simulink model "SPGF_FSK_0000_R2022b"  (R2022b)
settings: Solver=ode4  StartTime=0.0  StopTime=1.4  FixedStep=50e-6/50  RelTol=1e-3  EnableMultiTasking=on
undefined symbols (not defined in the file): D11, Delta
libraries: spsSeriesRLCBranchLib x1646, spsGroundLib x360, spsStairGeneratorLib x147, spsIdealSwitchLib x145, spsCurrentMeasurementLib x145, spsUniversalBridgeLib x76, spsThreePhaseSeriesRLCLoadLib x57, simulink x45, spsBistableLib x36, spsSequenceAnalyzerLib x31, spsThreePhaseParallelRLCLoadLib x20, spsThreePhaseTransformerTwoWindingsLib x20
(part 35 of 40)

== system SPGF_FSK_0000_R2022b/K2/fault/Arcing ==
  m : Inport
  Inter : Inport  Port=2
  Enable : EnablePort  StatesWhenEnabling=reset
  Abs3 : Abs  SaturateOnIntegerOverflow=off
  ArcStrV : Subsystem
  Bistable : spsBistableLib/Bistable  Qpriority=Set  ic=0  Ts=0
      settings: LibrarySourceBlock=sps_lib/Control/Bistable
  Constant1 : Constant  Value=TheoryOfArc
  Constant4 : Constant  Value=TheoryOfArc
  DTC_B : DataTypeConversion  OutDataTypeStr=boolean  SaturateOnIntegerOverflow=off  RndMeth=Floor
  DTC_D : DataTypeConversion  OutDataTypeStr=double  SaturateOnIntegerOverflow=off  RndMeth=Floor
  Demux : Demux  Outputs=2
  Fault A10 : Constant
  Fault A11 : Constant  Value=0
  Peters & Slepian : Subsystem
  Product : Product
  Relational Operator4 : RelationalOperator  OutDataTypeStr=boolean  InputSameDT=off
  SW_1 : MultiPortSwitch  DataPortForDefault=Additional data port  SaturateOnIntegerOverflow=off  InputSameDT=off
  SW_2 : Switch  Criteria=u2 > Threshold  Threshold=2  SaturateOnIntegerOverflow=off  InputSameDT=off
  Subsystem : Subsystem
  Terminator3 : Terminator
  Zero Crossing : Subsystem
  O : Outport  InitialOutput=[0]
  wires:
  Subsystem/1(O) -> Product/2
  Inter/1 -> [Inter]
  Relational Operator4/1 -> Product/1
  [Inter] -> Subsystem/1(I)
  Peters & Slepian/1(O) -> SW_2/1
  [I] -> Peters & Slepian/3(I)
  [Arc] -> Peters & Slepian/2(Arc)
  [I] -> Zero Crossing/1(I)
  Zero Crossing/1(O) -> SW_2/3, Peters & Slepian/1(ZC)  "Petersen"
  ArcStrV/1(Vset) -> Relational Operator4/2
  m/1 -> Demux/1
  Demux/2 -> [V]
  Demux/1 -> [I]
  Constant4/1 -> SW_2/2
  SW_2/1 -> DTC_B/1
  Abs3/1 -> Relational Operator4/1
  [V] -> Abs3/1
  DTC_D/1 -> SW_1/4, SW_1/3
  DTC_B/1 -> Bistable/2
  Bistable/2 -> Terminator3/1
  Product/1 -> [Arc], Bistable/1
  Bistable/1 -> DTC_D/1
  Fault A11/1 -> SW_1/5
  Fault A10/1 -> SW_1/2
  SW_1/1 -> O/1
  Constant1/1 -> SW_1/1

== system SPGF_FSK_0000_R2022b/K2/fault/Count Limiter ==
  I : Inport
  Counter : Subsystem  TreatAsAtomicUnit=on
  Fault A13 : Constant  Value=0
  Fault A3 : Constant
  Switch4 : Switch  Threshold=ArcingNumber  SaturateOnIntegerOverflow=off  InputSameDT=off
  Count : Outport
  O : Outport  Port=2
  wires:
  Counter/1(O) -> Count/1, Switch4/2
  Fault A13/1 -> Switch4/1
  Fault A3/1 -> Counter/1(I)
  I/1 -> Counter/Trigger, Switch4/3
  Switch4/1 -> O/1

== system SPGF_FSK_0000_R2022b/K2/fault/InitialPhaseCtrl ==
  m : Inport
  Enable : EnablePort  StatesWhenEnabling=reset
  Bistable : spsBistableLib/Bistable  Qpriority=Set  ic=0  Ts=0
      settings: LibrarySourceBlock=sps_lib/Control/Bistable
  Bistable1 : spsBistableLib/Bistable  Qpriority=Set  ic=0  Ts=0
      settings: LibrarySourceBlock=sps_lib/Control/Bistable
  Compare To Zero : simulink/Logic and Bit Operations/Compare To Zero  relop=~=  OutDataTypeStr=boolean
  Constant1 : Constant  Value=InitialPhaseCtrl
  DTC_D : DataTypeConversion  OutDataTypeStr=double  SaturateOnIntegerOverflow=off  RndMeth=Floor
  DTC_D1 : DataTypeConversion  OutDataTypeStr=double  SaturateOnIntegerOverflow=off  RndMeth=Floor
  DTC_D2 : DataTypeConversion  OutDataTypeStr=double  SaturateOnIntegerOverflow=off  RndMeth=Floor
  Demux : Demux  Outputs=2
  Fault A11 : Constant
  Hit Crossing : HitCross
  Off Delay : spsOffDelayLib/Off Delay  DelayType=On delay  delay=FaultDelay  ic=0  Ts=0
      settings: LibrarySourceBlock=sps_lib/Control/Off Delay
  Product1 : Product
  SW_1 : MultiPortSwitch  Inputs=2  SaturateOnIntegerOverflow=off  InputSameDT=off
  Terminator : Terminator
  Terminator1 : Terminator
  Terminator3 : Terminator
  O : Outport  InitialOutput=[0]
  wires:
  Bistable1/2 -> Terminator1/1
  DTC_D1/1 -> Product1/2
  Bistable1/1 -> DTC_D1/1
  DTC_D/1 -> SW_1/2
  Fault A11/1 -> SW_1/3
  Off Delay/1 -> Bistable/1
  Bistable/1 -> DTC_D/1
  Bistable/2 -> Terminator3/1
  Constant1/1 -> SW_1/1
  SW_1/1 -> O/1
  Demux/1 -> Terminator/1
  Demux/2 -> [V]
  m/1 -> Demux/1
  Product1/1 -> Off Delay/1
  [V] -> Hit Crossing/1, Compare To Zero/1
  Compare To Zero/1 -> DTC_D2/1
  Hit Crossing/1 -> Bistable1/1
  DTC_D2/1 -> Product1/1

== system SPGF_FSK_0000_R2022b/K2/fault/Interruption ==
  Band-Limited White Noise1 : simulink/Sources/Band-Limited White Noise  Cov=[.1]  Ts=NoiseSampleTime  seed=NoiseSeed
  Constant1 : Constant  Value=TypeOfPause
  Fault A10 : Constant
  Fault A11 : Constant  Value=0
  Multiport Switch : MultiPortSwitch  Inputs=4  DataPortForDefault=Additional data port  SaturateOnIntegerOverflow=off  InputSameDT=off
  Pulse Generator : DiscretePulseGenerator  PulseType=Time based  Period=PulsePeriod  PulseWidth=PulseWidth  PhaseDelay=PhaseDelay
  Rate Transition1 : RateTransition
  Saturation1 : Saturate  UpperLimit=1  LowerLimit=0
  Sign1 : Signum
  "Stair Generator " : spsStairGeneratorLib/Stair Generator  t=SwitchTimes  e=SwitchStatus  Ts=0
  O : Outport
  wires:
  Band-Limited White Noise1/1 -> Sign1/1
  "Stair Generator "/1 -> Multiport Switch/5
  Rate Transition1/1 -> Multiport Switch/3
  Saturation1/1 -> Rate Transition1/1
  Pulse Generator/1 -> Multiport Switch/4
  Constant1/1 -> Multiport Switch/1
  Sign1/1 -> Saturation1/1
  Fault A11/1 -> Multiport Switch/6
  Fault A10/1 -> Multiport Switch/2
  Multiport Switch/1 -> O/1

== system SPGF_FSK_0000_R2022b/K2/fault/Time Delay ==
  Count : Inport
  Control : Inport  Port=2
  Constant1 : Constant  Value=TimeDelay
  Constant3 : Constant  Value=0
  Memory : Memory
  SC_Time5 : Subsystem
      mask Display: disp('Delay');
  SW_Num : Switch  Threshold=ArcingNumber  SaturateOnIntegerOverflow=off  InputSameDT=off
  Selector : Selector  IndexMode=Zero-based  InputPortWidth=ArcingNumber  IndexOptions=Index vector (port)  Indices=[1 4]  OutputSizes=1
  O : Outport
  wires:
  Memory/1 -> SW_Num/3
  Control/1 -> SC_Time5/1(Control)
  SC_Time5/1(Out) -> O/1
  Count/1 -> SW_Num/2, Memory/1
  Constant1/1 -> Selector/1
  Selector/1 -> SC_Time5/2(TimeDelay)
  Constant3/1 -> SW_Num/1
  SW_Num/1 -> Selector/2

== system SPGF_FSK_0000_R2022b/K3/fault/Arcing ==
  m : Inport
  Inter : Inport  Port=2
  Enable : EnablePort  StatesWhenEnabling=reset
  Abs3 : Abs  SaturateOnIntegerOverflow=off
  ArcStrV : Subsystem
  Bistable : spsBistableLib/Bistable  Qpriority=Set  ic=0  Ts=0
      settings: LibrarySourceBlock=sps_lib/Control/Bistable
  Constant1 : Constant  Value=TheoryOfArc
  Constant4 : Constant  Value=TheoryOfArc
  DTC_B : DataTypeConversion  OutDataTypeStr=boolean  SaturateOnIntegerOverflow=off  RndMeth=Floor
  DTC_D : DataTypeConversion  OutDataTypeStr=double  SaturateOnIntegerOverflow=off  RndMeth=Floor
  Demux : Demux  Outputs=2
  Fault A10 : Constant
  Fault A11 : Constant  Value=0
  Peters & Slepian : Subsystem
  Product : Product
  Relational Operator4 : RelationalOperator  OutDataTypeStr=boolean  InputSameDT=off
  SW_1 : MultiPortSwitch  DataPortForDefault=Additional data port  SaturateOnIntegerOverflow=off  InputSameDT=off
  SW_2 : Switch  Criteria=u2 > Threshold  Threshold=2  SaturateOnIntegerOverflow=off  InputSameDT=off
  Subsystem : Subsystem
  Terminator3 : Terminator
  Zero Crossing : Subsystem
  O : Outport  InitialOutput=[0]
  wires:
  Subsystem/1(O) -> Product/2
  Inter/1 -> [Inter]
  Relational Operator4/1 -> Product/1
  [Inter] -> Subsystem/1(I)
  Peters & Slepian/1(O) -> SW_2/1
  [I] -> Peters & Slepian/3(I)
  [Arc] -> Peters & Slepian/2(Arc)
  [I] -> Zero Crossing/1(I)
  Zero Crossing/1(O) -> SW_2/3, Peters & Slepian/1(ZC)  "Petersen"
  ArcStrV/1(Vset) -> Relational Operator4/2
  m/1 -> Demux/1
  Demux/2 -> [V]
  Demux/1 -> [I]
  Constant4/1 -> SW_2/2
  SW_2/1 -> DTC_B/1
  Abs3/1 -> Relational Operator4/1
  [V] -> Abs3/1
  DTC_D/1 -> SW_1/4, SW_1/3
  DTC_B/1 -> Bistable/2
  Bistable/2 -> Terminator3/1
  Product/1 -> [Arc], Bistable/1
  Bistable/1 -> DTC_D/1
  Fault A11/1 -> SW_1/5
  Fault A10/1 -> SW_1/2
  SW_1/1 -> O/1
  Constant1/1 -> SW_1/1

== system SPGF_FSK_0000_R2022b/K3/fault/Count Limiter ==
  I : Inport
  Counter : Subsystem  TreatAsAtomicUnit=on
  Fault A13 : Constant  Value=0
  Fault A3 : Constant
  Switch4 : Switch  Threshold=ArcingNumber  SaturateOnIntegerOverflow=off  InputSameDT=off
  Count : Outport
  O : Outport  Port=2
  wires:
  Counter/1(O) -> Count/1, Switch4/2
  Fault A13/1 -> Switch4/1
  Fault A3/1 -> Counter/1(I)
  I/1 -> Counter/Trigger, Switch4/3
  Switch4/1 -> O/1

== system SPGF_FSK_0000_R2022b/K3/fault/InitialPhaseCtrl ==
  m : Inport
  Enable : EnablePort  StatesWhenEnabling=reset
  Bistable : spsBistableLib/Bistable  Qpriority=Set  ic=0  Ts=0
      settings: LibrarySourceBlock=sps_lib/Control/Bistable
  Bistable1 : spsBistableLib/Bistable  Qpriority=Set  ic=0  Ts=0
      settings: LibrarySourceBlock=sps_lib/Control/Bistable
  Compare To Zero : simulink/Logic and Bit Operations/Compare To Zero  relop=~=  OutDataTypeStr=boolean
  Constant1 : Constant  Value=InitialPhaseCtrl
  DTC_D : DataTypeConversion  OutDataTypeStr=double  SaturateOnIntegerOverflow=off  RndMeth=Floor
  DTC_D1 : DataTypeConversion  OutDataTypeStr=double  SaturateOnIntegerOverflow=off  RndMeth=Floor
  DTC_D2 : DataTypeConversion  OutDataTypeStr=double  SaturateOnIntegerOverflow=off  RndMeth=Floor
  Demux : Demux  Outputs=2
  Fault A11 : Constant
  Hit Crossing : HitCross
  Off Delay : spsOffDelayLib/Off Delay  DelayType=On delay  delay=FaultDelay  ic=0  Ts=0
      settings: LibrarySourceBlock=sps_lib/Control/Off Delay
  Product1 : Product
  SW_1 : MultiPortSwitch  Inputs=2  SaturateOnIntegerOverflow=off  InputSameDT=off
  Terminator : Terminator
  Terminator1 : Terminator
  Terminator3 : Terminator
  O : Outport  InitialOutput=[0]
  wires:
  Bistable1/2 -> Terminator1/1
  DTC_D1/1 -> Product1/2
  Bistable1/1 -> DTC_D1/1
  DTC_D/1 -> SW_1/2
  Fault A11/1 -> SW_1/3
  Off Delay/1 -> Bistable/1
  Bistable/1 -> DTC_D/1
  Bistable/2 -> Terminator3/1
  Constant1/1 -> SW_1/1
  SW_1/1 -> O/1
  Demux/1 -> Terminator/1
  Demux/2 -> [V]
  m/1 -> Demux/1
  Product1/1 -> Off Delay/1
  [V] -> Hit Crossing/1, Compare To Zero/1
  Compare To Zero/1 -> DTC_D2/1
  Hit Crossing/1 -> Bistable1/1
  DTC_D2/1 -> Product1/1

== system SPGF_FSK_0000_R2022b/K3/fault/Interruption ==
  Band-Limited White Noise1 : simulink/Sources/Band-Limited White Noise  Cov=[.1]  Ts=NoiseSampleTime  seed=NoiseSeed
  Constant1 : Constant  Value=TypeOfPause
  Fault A10 : Constant
  Fault A11 : Constant  Value=0
  Multiport Switch : MultiPortSwitch  Inputs=4  DataPortForDefault=Additional data port  SaturateOnIntegerOverflow=off  InputSameDT=off
  Pulse Generator : DiscretePulseGenerator  PulseType=Time based  Period=PulsePeriod  PulseWidth=PulseWidth  PhaseDelay=PhaseDelay
  Rate Transition1 : RateTransition
  Saturation1 : Saturate  UpperLimit=1  LowerLimit=0
  Sign1 : Signum
  "Stair Generator " : spsStairGeneratorLib/Stair Generator  t=SwitchTimes  e=SwitchStatus  Ts=0
  O : Outport
  wires:
  Band-Limited White Noise1/1 -> Sign1/1
  "Stair Generator "/1 -> Multiport Switch/5
  Rate Transition1/1 -> Multiport Switch/3
  Saturation1/1 -> Rate Transition1/1
  Pulse Generator/1 -> Multiport Switch/4
  Constant1/1 -> Multiport Switch/1
  Sign1/1 -> Saturation1/1
  Fault A11/1 -> Multiport Switch/6
  Fault A10/1 -> Multiport Switch/2
  Multiport Switch/1 -> O/1

== system SPGF_FSK_0000_R2022b/K3/fault/Time Delay ==
  Count : Inport
  Control : Inport  Port=2
  Constant1 : Constant  Value=TimeDelay
  Constant3 : Constant  Value=0
  Memory : Memory
  SC_Time5 : Subsystem
      mask Display: disp('Delay');
  SW_Num : Switch  Threshold=ArcingNumber  SaturateOnIntegerOverflow=off  InputSameDT=off
  Selector : Selector  IndexMode=Zero-based  InputPortWidth=ArcingNumber  IndexOptions=Index vector (port)  Indices=[1 4]  OutputSizes=1
  O : Outport
  wires:
  Memory/1 -> SW_Num/3
  Control/1 -> SC_Time5/1(Control)
  SC_Time5/1(Out) -> O/1
  Count/1 -> SW_Num/2, Memory/1
  Constant1/1 -> Selector/1
  Selector/1 -> SC_Time5/2(TimeDelay)
  Constant3/1 -> SW_Num/1
  SW_Num/1 -> Selector/2

== system SPGF_FSK_0000_R2022b/K4/fault/Arcing ==
  m : Inport
  Inter : Inport  Port=2
  Enable : EnablePort  StatesWhenEnabling=reset
  Abs3 : Abs  SaturateOnIntegerOverflow=off
  ArcStrV : Subsystem
  Bistable : spsBistableLib/Bistable  Qpriority=Set  ic=0  Ts=0
      settings: LibrarySourceBlock=sps_lib/Control/Bistable
  Constant1 : Constant  Value=TheoryOfArc
  Constant4 : Constant  Value=TheoryOfArc
  DTC_B : DataTypeConversion  OutDataTypeStr=boolean  SaturateOnIntegerOverflow=off  RndMeth=Floor
  DTC_D : DataTypeConversion  OutDataTypeStr=double  SaturateOnIntegerOverflow=off  RndMeth=Floor
  Demux : Demux  Outputs=2
  Fault A10 : Constant
  Fault A11 : Constant  Value=0
  Peters & Slepian : Subsystem
  Product : Product
  Relational Operator4 : RelationalOperator  OutDataTypeStr=boolean  InputSameDT=off
  SW_1 : MultiPortSwitch  DataPortForDefault=Additional data port  SaturateOnIntegerOverflow=off  InputSameDT=off
  SW_2 : Switch  Criteria=u2 > Threshold  Threshold=2  SaturateOnIntegerOverflow=off  InputSameDT=off
  Subsystem : Subsystem
  Terminator3 : Terminator
  Zero Crossing : Subsystem
  O : Outport  InitialOutput=[0]
  wires:
  Subsystem/1(O) -> Product/2
  Inter/1 -> [Inter]
  Relational Operator4/1 -> Product/1
  [Inter] -> Subsystem/1(I)
  Peters & Slepian/1(O) -> SW_2/1
  [I] -> Peters & Slepian/3(I)
  [Arc] -> Peters & Slepian/2(Arc)
  [I] -> Zero Crossing/1(I)
  Zero Crossing/1(O) -> SW_2/3, Peters & Slepian/1(ZC)  "Petersen"
  ArcStrV/1(Vset) -> Relational Operator4/2
  m/1 -> Demux/1
  Demux/2 -> [V]
  Demux/1 -> [I]
  Constant4/1 -> SW_2/2
  SW_2/1 -> DTC_B/1
  Abs3/1 -> Relational Operator4/1
  [V] -> Abs3/1
  DTC_D/1 -> SW_1/4, SW_1/3
  DTC_B/1 -> Bistable/2
  Bistable/2 -> Terminator3/1
  Product/1 -> [Arc], Bistable/1
  Bistable/1 -> DTC_D/1
  Fault A11/1 -> SW_1/5
  Fault A10/1 -> SW_1/2
  SW_1/1 -> O/1
  Constant1/1 -> SW_1/1

== system SPGF_FSK_0000_R2022b/K4/fault/Count Limiter ==
  I : Inport
  Counter : Subsystem  TreatAsAtomicUnit=on
  Fault A13 : Constant  Value=0
  Fault A3 : Constant
  Switch4 : Switch  Threshold=ArcingNumber  SaturateOnIntegerOverflow=off  InputSameDT=off
  Count : Outport
  O : Outport  Port=2
  wires:
  Counter/1(O) -> Count/1, Switch4/2
  Fault A13/1 -> Switch4/1
  Fault A3/1 -> Counter/1(I)
  I/1 -> Counter/Trigger, Switch4/3
  Switch4/1 -> O/1

== system SPGF_FSK_0000_R2022b/K4/fault/InitialPhaseCtrl ==
  m : Inport
  Enable : EnablePort  StatesWhenEnabling=reset
  Bistable : spsBistableLib/Bistable  Qpriority=Set  ic=0  Ts=0
      settings: LibrarySourceBlock=sps_lib/Control/Bistable
  Bistable1 : spsBistableLib/Bistable  Qpriority=Set  ic=0  Ts=0
      settings: LibrarySourceBlock=sps_lib/Control/Bistable
  Compare To Zero : simulink/Logic and Bit Operations/Compare To Zero  relop=~=  OutDataTypeStr=boolean
  Constant1 : Constant  Value=InitialPhaseCtrl
  DTC_D : DataTypeConversion  OutDataTypeStr=double  SaturateOnIntegerOverflow=off  RndMeth=Floor
  DTC_D1 : DataTypeConversion  OutDataTypeStr=double  SaturateOnIntegerOverflow=off  RndMeth=Floor
  DTC_D2 : DataTypeConversion  OutDataTypeStr=double  SaturateOnIntegerOverflow=off  RndMeth=Floor
  Demux : Demux  Outputs=2
  Fault A11 : Constant
  Hit Crossing : HitCross
  Off Delay : spsOffDelayLib/Off Delay  DelayType=On delay  delay=FaultDelay  ic=0  Ts=0
      settings: LibrarySourceBlock=sps_lib/Control/Off Delay
  Product1 : Product
  SW_1 : MultiPortSwitch  Inputs=2  SaturateOnIntegerOverflow=off  InputSameDT=off
  Terminator : Terminator
  Terminator1 : Terminator
  Terminator3 : Terminator
  O : Outport  InitialOutput=[0]
  wires:
  Bistable1/2 -> Terminator1/1
  DTC_D1/1 -> Product1/2
  Bistable1/1 -> DTC_D1/1
  DTC_D/1 -> SW_1/2
  Fault A11/1 -> SW_1/3
  Off Delay/1 -> Bistable/1
  Bistable/1 -> DTC_D/1
  Bistable/2 -> Terminator3/1
  Constant1/1 -> SW_1/1
  SW_1/1 -> O/1
  Demux/1 -> Terminator/1
  Demux/2 -> [V]
  m/1 -> Demux/1
  Product1/1 -> Off Delay/1
  [V] -> Hit Crossing/1, Compare To Zero/1
  Compare To Zero/1 -> DTC_D2/1
  Hit Crossing/1 -> Bistable1/1
  DTC_D2/1 -> Product1/1

== system SPGF_FSK_0000_R2022b/K4/fault/Interruption ==
  Band-Limited White Noise1 : simulink/Sources/Band-Limited White Noise  Cov=[.1]  Ts=NoiseSampleTime  seed=NoiseSeed
  Constant1 : Constant  Value=TypeOfPause
  Fault A10 : Constant
  Fault A11 : Constant  Value=0
  Multiport Switch : MultiPortSwitch  Inputs=4  DataPortForDefault=Additional data port  SaturateOnIntegerOverflow=off  InputSameDT=off
  Pulse Generator : DiscretePulseGenerator  PulseType=Time based  Period=PulsePeriod  PulseWidth=PulseWidth  PhaseDelay=PhaseDelay
  Rate Transition1 : RateTransition
  Saturation1 : Saturate  UpperLimit=1  LowerLimit=0
  Sign1 : Signum
  "Stair Generator " : spsStairGeneratorLib/Stair Generator  t=SwitchTimes  e=SwitchStatus  Ts=0
  O : Outport
  wires:
  Band-Limited White Noise1/1 -> Sign1/1
  "Stair Generator "/1 -> Multiport Switch/5
  Rate Transition1/1 -> Multiport Switch/3
  Saturation1/1 -> Rate Transition1/1
  Pulse Generator/1 -> Multiport Switch/4
  Constant1/1 -> Multiport Switch/1
  Sign1/1 -> Saturation1/1
  Fault A11/1 -> Multiport Switch/6
  Fault A10/1 -> Multiport Switch/2
  Multiport Switch/1 -> O/1

== system SPGF_FSK_0000_R2022b/K4/fault/Time Delay ==
  Count : Inport
  Control : Inport  Port=2
  Constant1 : Constant  Value=TimeDelay
  Constant3 : Constant  Value=0
  Memory : Memory
  SC_Time5 : Subsystem
      mask Display: disp('Delay');
  SW_Num : Switch  Threshold=ArcingNumber  SaturateOnIntegerOverflow=off  InputSameDT=off
  Selector : Selector  IndexMode=Zero-based  InputPortWidth=ArcingNumber  IndexOptions=Index vector (port)  Indices=[1 4]  OutputSizes=1
  O : Outport
  wires:
  Memory/1 -> SW_Num/3
  Control/1 -> SC_Time5/1(Control)
  SC_Time5/1(Out) -> O/1
  Count/1 -> SW_Num/2, Memory/1
  Constant1/1 -> Selector/1
  Selector/1 -> SC_Time5/2(TimeDelay)
  Constant3/1 -> SW_Num/1
  SW_Num/1 -> Selector/2

== system SPGF_FSK_0000_R2022b/K5/fault/Arcing ==
  m : Inport
  Inter : Inport  Port=2
  Enable : EnablePort  StatesWhenEnabling=reset
  Abs3 : Abs  SaturateOnIntegerOverflow=off
  ArcStrV : Subsystem
  Bistable : spsBistableLib/Bistable  Qpriority=Set  ic=0  Ts=0
      settings: LibrarySourceBlock=sps_lib/Control/Bistable
  Constant1 : Constant  Value=TheoryOfArc
  Constant4 : Constant  Value=TheoryOfArc
  DTC_B : DataTypeConversion  OutDataTypeStr=boolean  SaturateOnIntegerOverflow=off  RndMeth=Floor
  DTC_D : DataTypeConversion  OutDataTypeStr=double  SaturateOnIntegerOverflow=off  RndMeth=Floor
  Demux : Demux  Outputs=2
  Fault A10 : Constant
  Fault A11 : Constant  Value=0
  Peters & Slepian : Subsystem
  Product : Product
  Relational Operator4 : RelationalOperator  OutDataTypeStr=boolean  InputSameDT=off
  SW_1 : MultiPortSwitch  DataPortForDefault=Additional data port  SaturateOnIntegerOverflow=off  InputSameDT=off
  SW_2 : Switch  Criteria=u2 > Threshold  Threshold=2  SaturateOnIntegerOverflow=off  InputSameDT=off
  Subsystem : Subsystem
  Terminator3 : Terminator
  Zero Crossing : Subsystem
  O : Outport  InitialOutput=[0]
  wires:
  Subsystem/1(O) -> Product/2
  Inter/1 -> [Inter]
  Relational Operator4/1 -> Product/1
  [Inter] -> Subsystem/1(I)
  Peters & Slepian/1(O) -> SW_2/1
  [I] -> Peters & Slepian/3(I)
  [Arc] -> Peters & Slepian/2(Arc)
  [I] -> Zero Crossing/1(I)
  Zero Crossing/1(O) -> SW_2/3, Peters & Slepian/1(ZC)  "Petersen"
  ArcStrV/1(Vset) -> Relational Operator4/2
  m/1 -> Demux/1
  Demux/2 -> [V]
  Demux/1 -> [I]
  Constant4/1 -> SW_2/2
  SW_2/1 -> DTC_B/1
  Abs3/1 -> Relational Operator4/1
  [V] -> Abs3/1
  DTC_D/1 -> SW_1/4, SW_1/3
  DTC_B/1 -> Bistable/2
  Bistable/2 -> Terminator3/1
  Product/1 -> [Arc], Bistable/1
  Bistable/1 -> DTC_D/1
  Fault A11/1 -> SW_1/5
  Fault A10/1 -> SW_1/2
  SW_1/1 -> O/1
  Constant1/1 -> SW_1/1

== system SPGF_FSK_0000_R2022b/K5/fault/Count Limiter ==
  I : Inport
  Counter : Subsystem  TreatAsAtomicUnit=on
  Fault A13 : Constant  Value=0
  Fault A3 : Constant
  Switch4 : Switch  Threshold=ArcingNumber  SaturateOnIntegerOverflow=off  InputSameDT=off
  Count : Outport
  O : Outport  Port=2
  wires:
  Counter/1(O) -> Count/1, Switch4/2
  Fault A13/1 -> Switch4/1
  Fault A3/1 -> Counter/1(I)
  I/1 -> Counter/Trigger, Switch4/3
  Switch4/1 -> O/1

== system SPGF_FSK_0000_R2022b/K5/fault/InitialPhaseCtrl ==
  m : Inport
  Enable : EnablePort  StatesWhenEnabling=reset
  Bistable : spsBistableLib/Bistable  Qpriority=Set  ic=0  Ts=0
      settings: LibrarySourceBlock=sps_lib/Control/Bistable
  Bistable1 : spsBistableLib/Bistable  Qpriority=Set  ic=0  Ts=0
      settings: LibrarySourceBlock=sps_lib/Control/Bistable
  Compare To Zero : simulink/Logic and Bit Operations/Compare To Zero  relop=~=  OutDataTypeStr=boolean
  Constant1 : Constant  Value=InitialPhaseCtrl
  DTC_D : DataTypeConversion  OutDataTypeStr=double  SaturateOnIntegerOverflow=off  RndMeth=Floor
  DTC_D1 : DataTypeConversion  OutDataTypeStr=double  SaturateOnIntegerOverflow=off  RndMeth=Floor
  DTC_D2 : DataTypeConversion  OutDataTypeStr=double  SaturateOnIntegerOverflow=off  RndMeth=Floor
  Demux : Demux  Outputs=2
  Fault A11 : Constant
  Hit Crossing : HitCross
  Off Delay : spsOffDelayLib/Off Delay  DelayType=On delay  delay=FaultDelay  ic=0  Ts=0
      settings: LibrarySourceBlock=sps_lib/Control/Off Delay
  Product1 : Product
  SW_1 : MultiPortSwitch  Inputs=2  SaturateOnIntegerOverflow=off  InputSameDT=off
  Terminator : Terminator
  Terminator1 : Terminator
  Terminator3 : Terminator
  O : Outport  InitialOutput=[0]
  wires:
  Bistable1/2 -> Terminator1/1
  DTC_D1/1 -> Product1/2
  Bistable1/1 -> DTC_D1/1
  DTC_D/1 -> SW_1/2
  Fault A11/1 -> SW_1/3
  Off Delay/1 -> Bistable/1
  Bistable/1 -> DTC_D/1
  Bistable/2 -> Terminator3/1
  Constant1/1 -> SW_1/1
  SW_1/1 -> O/1
  Demux/1 -> Terminator/1
  Demux/2 -> [V]
  m/1 -> Demux/1
  Product1/1 -> Off Delay/1
  [V] -> Hit Crossing/1, Compare To Zero/1
  Compare To Zero/1 -> DTC_D2/1
  Hit Crossing/1 -> Bistable1/1
  DTC_D2/1 -> Product1/1

== system SPGF_FSK_0000_R2022b/K5/fault/Interruption ==
  Band-Limited White Noise1 : simulink/Sources/Band-Limited White Noise  Cov=[.1]  Ts=NoiseSampleTime  seed=NoiseSeed
  Constant1 : Constant  Value=TypeOfPause
  Fault A10 : Constant
  Fault A11 : Constant  Value=0
  Multiport Switch : MultiPortSwitch  Inputs=4  DataPortForDefault=Additional data port  SaturateOnIntegerOverflow=off  InputSameDT=off
  Pulse Generator : DiscretePulseGenerator  PulseType=Time based  Period=PulsePeriod  PulseWidth=PulseWidth  PhaseDelay=PhaseDelay
  Rate Transition1 : RateTransition
  Saturation1 : Saturate  UpperLimit=1  LowerLimit=0
  Sign1 : Signum
  "Stair Generator " : spsStairGeneratorLib/Stair Generator  t=SwitchTimes  e=SwitchStatus  Ts=0
  O : Outport
  wires:
  Band-Limited White Noise1/1 -> Sign1/1
  "Stair Generator "/1 -> Multiport Switch/5
  Rate Transition1/1 -> Multiport Switch/3
  Saturation1/1 -> Rate Transition1/1
  Pulse Generator/1 -> Multiport Switch/4
  Constant1/1 -> Multiport Switch/1
  Sign1/1 -> Saturation1/1
  Fault A11/1 -> Multiport Switch/6
  Fault A10/1 -> Multiport Switch/2
  Multiport Switch/1 -> O/1

== system SPGF_FSK_0000_R2022b/K5/fault/Time Delay ==
  Count : Inport
  Control : Inport  Port=2
  Constant1 : Constant  Value=TimeDelay
  Constant3 : Constant  Value=0
  Memory : Memory
  SC_Time5 : Subsystem
      mask Display: disp('Delay');
  SW_Num : Switch  Threshold=ArcingNumber  SaturateOnIntegerOverflow=off  InputSameDT=off
  Selector : Selector  IndexMode=Zero-based  InputPortWidth=ArcingNumber  IndexOptions=Index vector (port)  Indices=[1 4]  OutputSizes=1
  O : Outport
  wires:
  Memory/1 -> SW_Num/3
  Control/1 -> SC_Time5/1(Control)
  SC_Time5/1(Out) -> O/1
  Count/1 -> SW_Num/2, Memory/1
  Constant1/1 -> Selector/1
  Selector/1 -> SC_Time5/2(TimeDelay)
  Constant3/1 -> SW_Num/1
  SW_Num/1 -> Selector/2

== system SPGF_FSK_0000_R2022b/K6/fault/Arcing ==
  m : Inport
  Inter : Inport  Port=2
  Enable : EnablePort  StatesWhenEnabling=reset
  Abs3 : Abs  SaturateOnIntegerOverflow=off
  ArcStrV : Subsystem
  Bistable : spsBistableLib/Bistable  Qpriority=Set  ic=0  Ts=0
      settings: LibrarySourceBlock=sps_lib/Control/Bistable
  Constant1 : Constant  Value=TheoryOfArc
  Constant4 : Constant  Value=TheoryOfArc
  DTC_B : DataTypeConversion  OutDataTypeStr=boolean  SaturateOnIntegerOverflow=off  RndMeth=Floor
  DTC_D : DataTypeConversion  OutDataTypeStr=double  SaturateOnIntegerOverflow=off  RndMeth=Floor
  Demux : Demux  Outputs=2
  Fault A10 : Constant
  Fault A11 : Constant  Value=0
  Peters & Slepian : Subsystem
  Product : Product
  Relational Operator4 : RelationalOperator  OutDataTypeStr=boolean  InputSameDT=off
  SW_1 : MultiPortSwitch  DataPortForDefault=Additional data port  SaturateOnIntegerOverflow=off  InputSameDT=off
  SW_2 : Switch  Criteria=u2 > Threshold  Threshold=2  SaturateOnIntegerOverflow=off  InputSameDT=off
  Subsystem : Subsystem
  Terminator3 : Terminator
  Zero Crossing : Subsystem
  O : Outport  InitialOutput=[0]
  wires:
  Subsystem/1(O) -> Product/2
  Inter/1 -> [Inter]
  Relational Operator4/1 -> Product/1
  [Inter] -> Subsystem/1(I)
  Peters & Slepian/1(O) -> SW_2/1
  [I] -> Peters & Slepian/3(I)
  [Arc] -> Peters & Slepian/2(Arc)
  [I] -> Zero Crossing/1(I)
  Zero Crossing/1(O) -> SW_2/3, Peters & Slepian/1(ZC)  "Petersen"
  ArcStrV/1(Vset) -> Relational Operator4/2
  m/1 -> Demux/1
  Demux/2 -> [V]
  Demux/1 -> [I]
  Constant4/1 -> SW_2/2
  SW_2/1 -> DTC_B/1
  Abs3/1 -> Relational Operator4/1
  [V] -> Abs3/1
  DTC_D/1 -> SW_1/4, SW_1/3
  DTC_B/1 -> Bistable/2
  Bistable/2 -> Terminator3/1
  Product/1 -> [Arc], Bistable/1
  Bistable/1 -> DTC_D/1
  Fault A11/1 -> SW_1/5
  Fault A10/1 -> SW_1/2
  SW_1/1 -> O/1
  Constant1/1 -> SW_1/1

== system SPGF_FSK_0000_R2022b/K6/fault/Count Limiter ==
  I : Inport
  Counter : Subsystem  TreatAsAtomicUnit=on
  Fault A13 : Constant  Value=0
  Fault A3 : Constant
  Switch4 : Switch  Threshold=ArcingNumber  SaturateOnIntegerOverflow=off  InputSameDT=off
  Count : Outport
  O : Outport  Port=2
  wires:
  Counter/1(O) -> Count/1, Switch4/2
  Fault A13/1 -> Switch4/1
  Fault A3/1 -> Counter/1(I)
  I/1 -> Counter/Trigger, Switch4/3
  Switch4/1 -> O/1

== system SPGF_FSK_0000_R2022b/K6/fault/InitialPhaseCtrl ==
  m : Inport
  Enable : EnablePort  StatesWhenEnabling=reset
  Bistable : spsBistableLib/Bistable  Qpriority=Set  ic=0  Ts=0
      settings: LibrarySourceBlock=sps_lib/Control/Bistable
  Bistable1 : spsBistableLib/Bistable  Qpriority=Set  ic=0  Ts=0
      settings: LibrarySourceBlock=sps_lib/Control/Bistable
  Compare To Zero : simulink/Logic and Bit Operations/Compare To Zero  relop=~=  OutDataTypeStr=boolean
  Constant1 : Constant  Value=InitialPhaseCtrl
  DTC_D : DataTypeConversion  OutDataTypeStr=double  SaturateOnIntegerOverflow=off  RndMeth=Floor
  DTC_D1 : DataTypeConversion  OutDataTypeStr=double  SaturateOnIntegerOverflow=off  RndMeth=Floor
  DTC_D2 : DataTypeConversion  OutDataTypeStr=double  SaturateOnIntegerOverflow=off  RndMeth=Floor
  Demux : Demux  Outputs=2
  Fault A11 : Constant
  Hit Crossing : HitCross
  Off Delay : spsOffDelayLib/Off Delay  DelayType=On delay  delay=FaultDelay  ic=0  Ts=0
      settings: LibrarySourceBlock=sps_lib/Control/Off Delay
  Product1 : Product
  SW_1 : MultiPortSwitch  Inputs=2  SaturateOnIntegerOverflow=off  InputSameDT=off
  Terminator : Terminator
  Terminator1 : Terminator
  Terminator3 : Terminator
  O : Outport  InitialOutput=[0]
  wires:
  Bistable1/2 -> Terminator1/1
  DTC_D1/1 -> Product1/2
  Bistable1/1 -> DTC_D1/1
  DTC_D/1 -> SW_1/2
  Fault A11/1 -> SW_1/3
  Off Delay/1 -> Bistable/1
  Bistable/1 -> DTC_D/1
  Bistable/2 -> Terminator3/1
  Constant1/1 -> SW_1/1
  SW_1/1 -> O/1
  Demux/1 -> Terminator/1
  Demux/2 -> [V]
  m/1 -> Demux/1
  Product1/1 -> Off Delay/1
  [V] -> Hit Crossing/1, Compare To Zero/1
  Compare To Zero/1 -> DTC_D2/1
  Hit Crossing/1 -> Bistable1/1
  DTC_D2/1 -> Product1/1

== system SPGF_FSK_0000_R2022b/K6/fault/Interruption ==
  Band-Limited White Noise1 : simulink/Sources/Band-Limited White Noise  Cov=[.1]  Ts=NoiseSampleTime  seed=NoiseSeed
  Constant1 : Constant  Value=TypeOfPause
  Fault A10 : Constant
  Fault A11 : Constant  Value=0
  Multiport Switch : MultiPortSwitch  Inputs=4  DataPortForDefault=Additional data port  SaturateOnIntegerOverflow=off  InputSameDT=off
  Pulse Generator : DiscretePulseGenerator  PulseType=Time based  Period=PulsePeriod  PulseWidth=PulseWidth  PhaseDelay=PhaseDelay
  Rate Transition1 : RateTransition
  Saturation1 : Saturate  UpperLimit=1  LowerLimit=0
  Sign1 : Signum
  "Stair Generator " : spsStairGeneratorLib/Stair Generator  t=SwitchTimes  e=SwitchStatus  Ts=0
  O : Outport
  wires:
  Band-Limited White Noise1/1 -> Sign1/1
  "Stair Generator "/1 -> Multiport Switch/5
  Rate Transition1/1 -> Multiport Switch/3
  Saturation1/1 -> Rate Transition1/1
  Pulse Generator/1 -> Multiport Switch/4
  Constant1/1 -> Multiport Switch/1
  Sign1/1 -> Saturation1/1
  Fault A11/1 -> Multiport Switch/6
  Fault A10/1 -> Multiport Switch/2
  Multiport Switch/1 -> O/1

== system SPGF_FSK_0000_R2022b/K6/fault/Time Delay ==
  Count : Inport
  Control : Inport  Port=2
  Constant1 : Constant  Value=TimeDelay
  Constant3 : Constant  Value=0
  Memory : Memory
  SC_Time5 : Subsystem
      mask Display: disp('Delay');
  SW_Num : Switch  Threshold=ArcingNumber  SaturateOnIntegerOverflow=off  InputSameDT=off
  Selector : Selector  IndexMode=Zero-based  InputPortWidth=ArcingNumber  IndexOptions=Index vector (port)  Indices=[1 4]  OutputSizes=1
  O : Outport
  wires:
  Memory/1 -> SW_Num/3
  Control/1 -> SC_Time5/1(Control)
  SC_Time5/1(Out) -> O/1
  Count/1 -> SW_Num/2, Memory/1
  Constant1/1 -> Selector/1
  Selector/1 -> SC_Time5/2(TimeDelay)
  Constant3/1 -> SW_Num/1
  SW_Num/1 -> Selector/2

== system SPGF_FSK_0000_R2022b/K8/fault/Arcing ==
  m : Inport
  Inter : Inport  Port=2
  Enable : EnablePort  StatesWhenEnabling=reset
  Abs3 : Abs  SaturateOnIntegerOverflow=off
  ArcStrV : Subsystem
  Bistable : spsBistableLib/Bistable  Qpriority=Set  ic=0  Ts=0
      settings: LibrarySourceBlock=sps_lib/Control/Bistable
  Constant1 : Constant  Value=TheoryOfArc
  Constant4 : Constant  Value=TheoryOfArc
  DTC_B : DataTypeConversion  OutDataTypeStr=boolean  SaturateOnIntegerOverflow=off  RndMeth=Floor
  DTC_D : DataTypeConversion  OutDataTypeStr=double  SaturateOnIntegerOverflow=off  RndMeth=Floor
  Demux : Demux  Outputs=2
  Fault A10 : Constant
  Fault A11 : Constant  Value=0
  Peters & Slepian : Subsystem
  Product : Product
  Relational Operator4 : RelationalOperator  OutDataTypeStr=boolean  InputSameDT=off
  SW_1 : MultiPortSwitch  DataPortForDefault=Additional data port  SaturateOnIntegerOverflow=off  InputSameDT=off
  SW_2 : Switch  Criteria=u2 > Threshold  Threshold=2  SaturateOnIntegerOverflow=off  InputSameDT=off
  Subsystem : Subsystem
  Terminator3 : Terminator
  Zero Crossing : Subsystem
  O : Outport  InitialOutput=[0]
  wires:
  Subsystem/1(O) -> Product/2
  Inter/1 -> [Inter]
  Relational Operator4/1 -> Product/1
  [Inter] -> Subsystem/1(I)
  Peters & Slepian/1(O) -> SW_2/1
  [I] -> Peters & Slepian/3(I)
  [Arc] -> Peters & Slepian/2(Arc)
  [I] -> Zero Crossing/1(I)
  Zero Crossing/1(O) -> SW_2/3, Peters & Slepian/1(ZC)  "Petersen"
  ArcStrV/1(Vset) -> Relational Operator4/2
  m/1 -> Demux/1
  Demux/2 -> [V]
  Demux/1 -> [I]
  Constant4/1 -> SW_2/2
  SW_2/1 -> DTC_B/1
  Abs3/1 -> Relational Operator4/1
  [V] -> Abs3/1
  DTC_D/1 -> SW_1/4, SW_1/3
  DTC_B/1 -> Bistable/2
  Bistable/2 -> Terminator3/1
  Product/1 -> [Arc], Bistable/1
  Bistable/1 -> DTC_D/1
  Fault A11/1 -> SW_1/5
  Fault A10/1 -> SW_1/2
  SW_1/1 -> O/1
  Constant1/1 -> SW_1/1

== system SPGF_FSK_0000_R2022b/K8/fault/Count Limiter ==
  I : Inport
  Counter : Subsystem  TreatAsAtomicUnit=on
  Fault A13 : Constant  Value=0
  Fault A3 : Constant
  Switch4 : Switch  Threshold=ArcingNumber  SaturateOnIntegerOverflow=off  InputSameDT=off
  Count : Outport
  O : Outport  Port=2
  wires:
  Counter/1(O) -> Count/1, Switch4/2
  Fault A13/1 -> Switch4/1
  Fault A3/1 -> Counter/1(I)
  I/1 -> Counter/Trigger, Switch4/3
  Switch4/1 -> O/1

== system SPGF_FSK_0000_R2022b/K8/fault/InitialPhaseCtrl ==
  m : Inport
  Enable : EnablePort  StatesWhenEnabling=reset
  Bistable : spsBistableLib/Bistable  Qpriority=Set  ic=0  Ts=0
      settings: LibrarySourceBlock=sps_lib/Control/Bistable
  Bistable1 : spsBistableLib/Bistable  Qpriority=Set  ic=0  Ts=0
      settings: LibrarySourceBlock=sps_lib/Control/Bistable
  Compare To Zero : simulink/Logic and Bit Operations/Compare To Zero  relop=~=  OutDataTypeStr=boolean
  Constant1 : Constant  Value=InitialPhaseCtrl
  DTC_D : DataTypeConversion  OutDataTypeStr=double  SaturateOnIntegerOverflow=off  RndMeth=Floor
  DTC_D1 : DataTypeConversion  OutDataTypeStr=double  SaturateOnIntegerOverflow=off  RndMeth=Floor
  DTC_D2 : DataTypeConversion  OutDataTypeStr=double  SaturateOnIntegerOverflow=off  RndMeth=Floor
  Demux : Demux  Outputs=2
  Fault A11 : Constant
  Hit Crossing : HitCross
  Off Delay : spsOffDelayLib/Off Delay  DelayType=On delay  delay=FaultDelay  ic=0  Ts=0
      settings: LibrarySourceBlock=sps_lib/Control/Off Delay
  Product1 : Product
  SW_1 : MultiPortSwitch  Inputs=2  SaturateOnIntegerOverflow=off  InputSameDT=off
  Terminator : Terminator
  Terminator1 : Terminator
  Terminator3 : Terminator
  O : Outport  InitialOutput=[0]
  wires:
  Bistable1/2 -> Terminator1/1
  DTC_D1/1 -> Product1/2
  Bistable1/1 -> DTC_D1/1
  DTC_D/1 -> SW_1/2
  Fault A11/1 -> SW_1/3
  Off Delay/1 -> Bistable/1
  Bistable/1 -> DTC_D/1
  Bistable/2 -> Terminator3/1
  Constant1/1 -> SW_1/1
  SW_1/1 -> O/1
  Demux/1 -> Terminator/1
  Demux/2 -> [V]
  m/1 -> Demux/1
  Product1/1 -> Off Delay/1
  [V] -> Hit Crossing/1, Compare To Zero/1
  Compare To Zero/1 -> DTC_D2/1
  Hit Crossing/1 -> Bistable1/1
  DTC_D2/1 -> Product1/1

== system SPGF_FSK_0000_R2022b/K8/fault/Interruption ==
  Band-Limited White Noise1 : simulink/Sources/Band-Limited White Noise  Cov=[.1]  Ts=NoiseSampleTime  seed=NoiseSeed
  Constant1 : Constant  Value=TypeOfPause
  Fault A10 : Constant
  Fault A11 : Constant  Value=0
  Multiport Switch : MultiPortSwitch  Inputs=4  DataPortForDefault=Additional data port  SaturateOnIntegerOverflow=off  InputSameDT=off
  Pulse Generator : DiscretePulseGenerator  PulseType=Time based  Period=PulsePeriod  PulseWidth=PulseWidth  PhaseDelay=PhaseDelay
  Rate Transition1 : RateTransition
  Saturation1 : Saturate  UpperLimit=1  LowerLimit=0
  Sign1 : Signum
  "Stair Generator " : spsStairGeneratorLib/Stair Generator  t=SwitchTimes  e=SwitchStatus  Ts=0
  O : Outport
  wires:
  Band-Limited White Noise1/1 -> Sign1/1
  "Stair Generator "/1 -> Multiport Switch/5
  Rate Transition1/1 -> Multiport Switch/3
  Saturation1/1 -> Rate Transition1/1
  Pulse Generator/1 -> Multiport Switch/4
  Constant1/1 -> Multiport Switch/1
  Sign1/1 -> Saturation1/1
  Fault A11/1 -> Multiport Switch/6
  Fault A10/1 -> Multiport Switch/2
  Multiport Switch/1 -> O/1

== system SPGF_FSK_0000_R2022b/K8/fault/Time Delay ==
  Count : Inport
  Control : Inport  Port=2
  Constant1 : Constant  Value=TimeDelay
  Constant3 : Constant  Value=0
  Memory : Memory
  SC_Time5 : Subsystem
      mask Display: disp('Delay');
  SW_Num : Switch  Threshold=ArcingNumber  SaturateOnIntegerOverflow=off  InputSameDT=off
  Selector : Selector  IndexMode=Zero-based  InputPortWidth=ArcingNumber  IndexOptions=Index vector (port)  Indices=[1 4]  OutputSizes=1
  O : Outport
  wires:
  Memory/1 -> SW_Num/3
  Control/1 -> SC_Time5/1(Control)
  SC_Time5/1(Out) -> O/1
  Count/1 -> SW_Num/2, Memory/1
  Constant1/1 -> Selector/1
  Selector/1 -> SC_Time5/2(TimeDelay)
  Constant3/1 -> SW_Num/1
  SW_Num/1 -> Selector/2

== system SPGF_FSK_0000_R2022b/K9/fault/Arcing ==
  m : Inport
  Inter : Inport  Port=2
  Enable : EnablePort  StatesWhenEnabling=reset
  Abs3 : Abs  SaturateOnIntegerOverflow=off
  ArcStrV : Subsystem
  Bistable : spsBistableLib/Bistable  Qpriority=Set  ic=0  Ts=0
      settings: LibrarySourceBlock=sps_lib/Control/Bistable
  Constant1 : Constant  Value=TheoryOfArc
  Constant4 : Constant  Value=TheoryOfArc
  DTC_B : DataTypeConversion  OutDataTypeStr=boolean  SaturateOnIntegerOverflow=off  RndMeth=Floor
  DTC_D : DataTypeConversion  OutDataTypeStr=double  SaturateOnIntegerOverflow=off  RndMeth=Floor
  Demux : Demux  Outputs=2
  Fault A10 : Constant
  Fault A11 : Constant  Value=0
  Peters & Slepian : Subsystem
  Product : Product
  Relational Operator4 : RelationalOperator  OutDataTypeStr=boolean  InputSameDT=off
  SW_1 : MultiPortSwitch  DataPortForDefault=Additional data port  SaturateOnIntegerOverflow=off  InputSameDT=off
  SW_2 : Switch  Criteria=u2 > Threshold  Threshold=2  SaturateOnIntegerOverflow=off  InputSameDT=off
  Subsystem : Subsystem
  Terminator3 : Terminator
  Zero Crossing : Subsystem
  O : Outport  InitialOutput=[0]
  wires:
  Subsystem/1(O) -> Product/2
  Inter/1 -> [Inter]
  Relational Operator4/1 -> Product/1
  [Inter] -> Subsystem/1(I)
  Peters & Slepian/1(O) -> SW_2/1
  [I] -> Peters & Slepian/3(I)
  [Arc] -> Peters & Slepian/2(Arc)
  [I] -> Zero Crossing/1(I)
  Zero Crossing/1(O) -> SW_2/3, Peters & Slepian/1(ZC)  "Petersen"
  ArcStrV/1(Vset) -> Relational Operator4/2
  m/1 -> Demux/1
  Demux/2 -> [V]
  Demux/1 -> [I]
  Constant4/1 -> SW_2/2
  SW_2/1 -> DTC_B/1
  Abs3/1 -> Relational Operator4/1
  [V] -> Abs3/1
  DTC_D/1 -> SW_1/4, SW_1/3
  DTC_B/1 -> Bistable/2
  Bistable/2 -> Terminator3/1
  Product/1 -> [Arc], Bistable/1
  Bistable/1 -> DTC_D/1
  Fault A11/1 -> SW_1/5
  Fault A10/1 -> SW_1/2
  SW_1/1 -> O/1
  Constant1/1 -> SW_1/1

== system SPGF_FSK_0000_R2022b/K9/fault/Count Limiter ==
  I : Inport
  Counter : Subsystem  TreatAsAtomicUnit=on
  Fault A13 : Constant  Value=0
  Fault A3 : Constant
  Switch4 : Switch  Threshold=ArcingNumber  SaturateOnIntegerOverflow=off  InputSameDT=off
  Count : Outport
  O : Outport  Port=2
  wires:
  Counter/1(O) -> Count/1, Switch4/2
  Fault A13/1 -> Switch4/1
  Fault A3/1 -> Counter/1(I)
  I/1 -> Counter/Trigger, Switch4/3
  Switch4/1 -> O/1

== system SPGF_FSK_0000_R2022b/K9/fault/InitialPhaseCtrl ==
  m : Inport
  Enable : EnablePort  StatesWhenEnabling=reset
  Bistable : spsBistableLib/Bistable  Qpriority=Set  ic=0  Ts=0
      settings: LibrarySourceBlock=sps_lib/Control/Bistable
  Bistable1 : spsBistableLib/Bistable  Qpriority=Set  ic=0  Ts=0
      settings: LibrarySourceBlock=sps_lib/Control/Bistable
  Compare To Zero : simulink/Logic and Bit Operations/Compare To Zero  relop=~=  OutDataTypeStr=boolean
  Constant1 : Constant  Value=InitialPhaseCtrl
  DTC_D : DataTypeConversion  OutDataTypeStr=double  SaturateOnIntegerOverflow=off  RndMeth=Floor
  DTC_D1 : DataTypeConversion  OutDataTypeStr=double  SaturateOnIntegerOverflow=off  RndMeth=Floor
  DTC_D2 : DataTypeConversion  OutDataTypeStr=double  SaturateOnIntegerOverflow=off  RndMeth=Floor
  Demux : Demux  Outputs=2
  Fault A11 : Constant
  Hit Crossing : HitCross
  Off Delay : spsOffDelayLib/Off Delay  DelayType=On delay  delay=FaultDelay  ic=0  Ts=0
      settings: LibrarySourceBlock=sps_lib/Control/Off Delay
  Product1 : Product
  SW_1 : MultiPortSwitch  Inputs=2  SaturateOnIntegerOverflow=off  InputSameDT=off
  Terminator : Terminator
  Terminator1 : Terminator
  Terminator3 : Terminator
  O : Outport  InitialOutput=[0]
  wires:
  Bistable1/2 -> Terminator1/1
  DTC_D1/1 -> Product1/2
  Bistable1/1 -> DTC_D1/1
  DTC_D/1 -> SW_1/2
  Fault A11/1 -> SW_1/3
  Off Delay/1 -> Bistable/1
  Bistable/1 -> DTC_D/1
  Bistable/2 -> Terminator3/1
  Constant1/1 -> SW_1/1
  SW_1/1 -> O/1
  Demux/1 -> Terminator/1
  Demux/2 -> [V]
  m/1 -> Demux/1
  Product1/1 -> Off Delay/1
  [V] -> Hit Crossing/1, Compare To Zero/1
  Compare To Zero/1 -> DTC_D2/1
  Hit Crossing/1 -> Bistable1/1
  DTC_D2/1 -> Product1/1

== system SPGF_FSK_0000_R2022b/K9/fault/Interruption ==
  Band-Limited White Noise1 : simulink/Sources/Band-Limited White Noise  Cov=[.1]  Ts=NoiseSampleTime  seed=NoiseSeed
  Constant1 : Constant  Value=TypeOfPause
  Fault A10 : Constant
  Fault A11 : Constant  Value=0
  Multiport Switch : MultiPortSwitch  Inputs=4  DataPortForDefault=Additional data port  SaturateOnIntegerOverflow=off  InputSameDT=off
  Pulse Generator : DiscretePulseGenerator  PulseType=Time based  Period=PulsePeriod  PulseWidth=PulseWidth  PhaseDelay=PhaseDelay
  Rate Transition1 : RateTransition
  Saturation1 : Saturate  UpperLimit=1  LowerLimit=0
  Sign1 : Signum
  "Stair Generator " : spsStairGeneratorLib/Stair Generator  t=SwitchTimes  e=SwitchStatus  Ts=0
  O : Outport
  wires:
  Band-Limited White Noise1/1 -> Sign1/1
  "Stair Generator "/1 -> Multiport Switch/5
  Rate Transition1/1 -> Multiport Switch/3
  Saturation1/1 -> Rate Transition1/1
  Pulse Generator/1 -> Multiport Switch/4
  Constant1/1 -> Multiport Switch/1
  Sign1/1 -> Saturation1/1
  Fault A11/1 -> Multiport Switch/6
  Fault A10/1 -> Multiport Switch/2
  Multiport Switch/1 -> O/1

== system SPGF_FSK_0000_R2022b/K9/fault/Time Delay ==
  Count : Inport
  Control : Inport  Port=2
  Constant1 : Constant  Value=TimeDelay
  Constant3 : Constant  Value=0
  Memory : Memory
  SC_Time5 : Subsystem
      mask Display: disp('Delay');
  SW_Num : Switch  Threshold=ArcingNumber  SaturateOnIntegerOverflow=off  InputSameDT=off
  Selector : Selector  IndexMode=Zero-based  InputPortWidth=ArcingNumber  IndexOptions=Index vector (port)  Indices=[1 4]  OutputSizes=1
  O : Outport
  wires:
  Memory/1 -> SW_Num/3
  Control/1 -> SC_Time5/1(Control)
  SC_Time5/1(Out) -> O/1
  Count/1 -> SW_Num/2, Memory/1
  Constant1/1 -> Selector/1
  Selector/1 -> SC_Time5/2(TimeDelay)
  Constant3/1 -> SW_Num/1
  SW_Num/1 -> Selector/2

== system SPGF_FSK_0000_R2022b/TP11/Q/breaker ==
  Fault A2 : Constant  Value=InitialStatus(3)
  Fault A3 : Constant  Value=InitialStatus(2)
  Fault A4 : Constant  Value=InitialStatus(1)
  Fault C1 : Constant  Value=SwitchC
  Fault C2 : Constant  Value=SwitchB
  Fault C3 : Constant  Value=SwitchA
  Ideal Switch A : spsIdealSwitchLib/Ideal Switch  Ron=BreakerResistance  Lon=0  IC=InitialStatus(1)  Rs=SnubberResistance  Cs=SnubberCapacitance  Measurements=off
  Ideal Switch B : spsIdealSwitchLib/Ideal Switch  Ron=BreakerResistance  Lon=0  IC=InitialStatus(2)  Rs=SnubberResistance  Cs=SnubberCapacitance  Measurements=off
  Ideal Switch C : spsIdealSwitchLib/Ideal Switch  Ron=BreakerResistance  Lon=0  IC=InitialStatus(3)  Rs=SnubberResistance  Cs=SnubberCapacitance  Measurements=off
  Stair Generator A : spsStairGeneratorLib/Stair Generator  t=SwitchTimesA  e=SwitchStatusA  Ts=0
  Stair Generator B : spsStairGeneratorLib/Stair Generator  t=SwitchTimesB  e=SwitchStatusB  Ts=0
  Stair Generator C : spsStairGeneratorLib/Stair Generator  t=SwitchTimesB  e=SwitchStatusB  Ts=0
  Switch2 : Switch  Criteria=u2 > Threshold  Threshold=0.5  SaturateOnIntegerOverflow=off  InputSameDT=off
  Switch3 : Switch  Criteria=u2 > Threshold  Threshold=0.5  SaturateOnIntegerOverflow=off  InputSameDT=off
  Switch4 : Switch  Criteria=u2 > Threshold  Threshold=0.5  SaturateOnIntegerOverflow=off  InputSameDT=off
  A : PMIOPort  Side=Left
  B : PMIOPort  Port=2  Side=Left
  C : PMIOPort  Port=3  Side=Left
  a : PMIOPort  Port=4  Side=Right
  b : PMIOPort  Port=5  Side=Right
  c : PMIOPort  Port=6  Side=Right
  wires:
  Switch2/1 -> Ideal Switch C/1
  Fault A2/1 -> Switch2/3
  Fault C1/1 -> Switch2/2
  Switch3/1 -> Ideal Switch B/1
  Fault A3/1 -> Switch3/3
  Fault C2/1 -> Switch3/2
  Fault A4/1 -> Switch4/3
  Fault C3/1 -> Switch4/2
  Switch4/1 -> Ideal Switch A/1
  Stair Generator B/1 -> Switch3/1
  Stair Generator A/1 -> Switch4/1
  Stair Generator C/1 -> Switch2/1
  connections:
  Ideal Switch B/LConn1 -- B/RConn1
  Ideal Switch A/LConn1 -- A/RConn1
  Ideal Switch C/LConn1 -- C/RConn1
  Ideal Switch A/RConn1 -- a/RConn1
  b/RConn1 -- Ideal Switch B/RConn1
  c/RConn1 -- Ideal Switch C/RConn1

== system SPGF_FSK_0000_R2022b/TP11/Q/meas ==
  Add : Sum  Inputs=+++
  GainI : Gain
  GainI0 : Gain
  I A: : spsCurrentMeasurementLib/Current Measurement  PhasorSimulation=off  OutputType=Complex  PSBequivalent=0
  I B: : spsCurrentMeasurementLib/Current Measurement  PhasorSimulation=off  OutputType=Complex  PSBequivalent=0
  I C: : spsCurrentMeasurementLib/Current Measurement  PhasorSimulation=off  OutputType=Complex  PSBequivalent=0
  Mux : Mux  Inputs=3
  A : PMIOPort  Side=Left
  B : PMIOPort  Port=2  Side=Left
  C : PMIOPort  Port=3  Side=Left
  a : PMIOPort  Port=4  Side=Right
  b : PMIOPort  Port=5  Side=Right
  c : PMIOPort  Port=6  Side=Right
  tag scope: CT3I0_TP11=global, CTIabc_TP11=global
  wires:
  I A:/1 -> Mux/1, Add/1
  I B:/1 -> Mux/2, Add/2
  I C:/1 -> Mux/3, Add/3
  Add/1 -> GainI0/1
  GainI0/1 -> [CT3I0_TP11]
  Mux/1 -> GainI/1
  GainI/1 -> [CTIabc_TP11]
  connections:
  I C:/RConn1 -- c/RConn1
  I B:/RConn1 -- b/RConn1
  a/RConn1 -- I A:/RConn1
  I A:/LConn1 -- A/RConn1
  I C:/LConn1 -- C/RConn1
  I B:/LConn1 -- B/RConn1

== system SPGF_FSK_0000_R2022b/TP11/Q/shunt ==
  A : PMIOPort  Side=Left
  B : PMIOPort  Port=2  Side=Left
  C : PMIOPort  Port=3  Side=Left
  a : PMIOPort  Port=4  Side=Right
  b : PMIOPort  Port=5  Side=Right
  c : PMIOPort  Port=6  Side=Right
  connections:
  C/RConn1 -- c/RConn1
  B/RConn1 -- b/RConn1
  A/RConn1 -- a/RConn1

== system SPGF_FSK_0000_R2022b/TP12/Q/breaker ==
  Fault A2 : Constant  Value=InitialStatus(3)
  Fault A3 : Constant  Value=InitialStatus(2)
  Fault A4 : Constant  Value=InitialStatus(1)
  Fault C1 : Constant  Value=SwitchC
  Fault C2 : Constant  Value=SwitchB
  Fault C3 : Constant  Value=SwitchA
  Ideal Switch A : spsIdealSwitchLib/Ideal Switch  Ron=BreakerResistance  Lon=0  IC=InitialStatus(1)  Rs=SnubberResistance  Cs=SnubberCapacitance  Measurements=off
  Ideal Switch B : spsIdealSwitchLib/Ideal Switch  Ron=BreakerResistance  Lon=0  IC=InitialStatus(2)  Rs=SnubberResistance  Cs=SnubberCapacitance  Measurements=off
  Ideal Switch C : spsIdealSwitchLib/Ideal Switch  Ron=BreakerResistance  Lon=0  IC=InitialStatus(3)  Rs=SnubberResistance  Cs=SnubberCapacitance  Measurements=off
  Stair Generator A : spsStairGeneratorLib/Stair Generator  t=SwitchTimesA  e=SwitchStatusA  Ts=0
  Stair Generator B : spsStairGeneratorLib/Stair Generator  t=SwitchTimesB  e=SwitchStatusB  Ts=0
  Stair Generator C : spsStairGeneratorLib/Stair Generator  t=SwitchTimesB  e=SwitchStatusB  Ts=0
  Switch2 : Switch  Criteria=u2 > Threshold  Threshold=0.5  SaturateOnIntegerOverflow=off  InputSameDT=off
  Switch3 : Switch  Criteria=u2 > Threshold  Threshold=0.5  SaturateOnIntegerOverflow=off  InputSameDT=off
  Switch4 : Switch  Criteria=u2 > Threshold  Threshold=0.5  SaturateOnIntegerOverflow=off  InputSameDT=off
  A : PMIOPort  Side=Left
  B : PMIOPort  Port=2  Side=Left
  C : PMIOPort  Port=3  Side=Left
  a : PMIOPort  Port=4  Side=Right
  b : PMIOPort  Port=5  Side=Right
  c : PMIOPort  Port=6  Side=Right
  wires:
  Switch2/1 -> Ideal Switch C/1
  Fault A2/1 -> Switch2/3
  Fault C1/1 -> Switch2/2
  Switch3/1 -> Ideal Switch B/1
  Fault A3/1 -> Switch3/3
  Fault C2/1 -> Switch3/2
  Fault A4/1 -> Switch4/3
  Fault C3/1 -> Switch4/2
  Switch4/1 -> Ideal Switch A/1
  Stair Generator B/1 -> Switch3/1
  Stair Generator A/1 -> Switch4/1
  Stair Generator C/1 -> Switch2/1
  connections:
  Ideal Switch B/LConn1 -- B/RConn1
  Ideal Switch A/LConn1 -- A/RConn1
  Ideal Switch C/LConn1 -- C/RConn1
  Ideal Switch A/RConn1 -- a/RConn1
  b/RConn1 -- Ideal Switch B/RConn1
  c/RConn1 -- Ideal Switch C/RConn1

== system SPGF_FSK_0000_R2022b/TP12/Q/meas ==
  Add : Sum  Inputs=+++
  GainI : Gain
  GainI0 : Gain
  I A: : spsCurrentMeasurementLib/Current Measurement  PhasorSimulation=off  OutputType=Complex  PSBequivalent=0
  I B: : spsCurrentMeasurementLib/Current Measurement  PhasorSimulation=off  OutputType=Complex  PSBequivalent=0
  I C: : spsCurrentMeasurementLib/Current Measurement  PhasorSimulation=off  OutputType=Complex  PSBequivalent=0
  Mux : Mux  Inputs=3
  A : PMIOPort  Side=Left
  B : PMIOPort  Port=2  Side=Left
  C : PMIOPort  Port=3  Side=Left
  a : PMIOPort  Port=4  Side=Right
  b : PMIOPort  Port=5  Side=Right
  c : PMIOPort  Port=6  Side=Right
  tag scope: CT3I0_TP12=global, CTIabc_TP12=global
  wires:
  I A:/1 -> Mux/1, Add/1
  I B:/1 -> Mux/2, Add/2
  I C:/1 -> Mux/3, Add/3
  Add/1 -> GainI0/1
  GainI0/1 -> [CT3I0_TP12]
  Mux/1 -> GainI/1
  GainI/1 -> [CTIabc_TP12]
  connections:
  I C:/RConn1 -- c/RConn1
  I B:/RConn1 -- b/RConn1
  a/RConn1 -- I A:/RConn1
  I A:/LConn1 -- A/RConn1
  I C:/LConn1 -- C/RConn1
  I B:/LConn1 -- B/RConn1

== system SPGF_FSK_0000_R2022b/TP12/Q/shunt ==
  A : PMIOPort  Side=Left
  B : PMIOPort  Port=2  Side=Left
  C : PMIOPort  Port=3  Side=Left
  a : PMIOPort  Port=4  Side=Right
  b : PMIOPort  Port=5  Side=Right
  c : PMIOPort  Port=6  Side=Right
  connections:
  C/RConn1 -- c/RConn1
  B/RConn1 -- b/RConn1
  A/RConn1 -- a/RConn1
